simulink model "Heli2DoF"  (R2024b)
settings: Solver=VariableStepAuto  StartTime=0.0  StopTime=30  RelTol=1e-3
values from neighbouring files (symbols this model uses):
  A = [0 0 1 0; 0 0 0 1; pp_ss.A(2,1) 0 pp_ss.A(2,2) 0; 0 0 0 yy_ss.A(2,2)]    [HeliControl.m]    (also in heli.mat = [0 0 -1.26336469915 0 0 0 0 0 1 0 -0.543659539999 0 ... (16 )
  B = [pp_ss.B(1,1) 0; yp_ss.B(1,1) 0; pp_ss.B(2,1) 0; 0 yy_ss.B(2,1)]    [HeliControl.m]    (also in heli.mat = [0.0358066695789  0; 0.0354869266893  0; 0.022302435285  0; )
  C = [1 0 0 0; 0 1 0 0]    [HeliControl.m]    (also in heli.mat = [1  0  0  0; 0  1  0  0])
  K = Ks(:,1:4)    [HeliControl.m]    (also in heli.mat = [45.6610986225  20.6092759277  20.0236061253  7.57450439059;)
  K_q = Kq(:,1:4)    [HeliControl.m]    (also in heli.mat = [20.1841001288  13.9498910139  11.326144531  5.03030863759; )
  Ki = -Ks(:,5:6)    [HeliControl.m]    (also in heli.mat = [18.7111763277  13.9796595605; 21.5110334967  -19.8867838349)
  Ki_q = -Kq(:,5:6)    [HeliControl.m]    (also in heli.mat = [19.1284159126  11.5803153962; 23.1606307923  -38.2568318252)
settings Model: Creator=nagel  LastModifiedBy=nagel

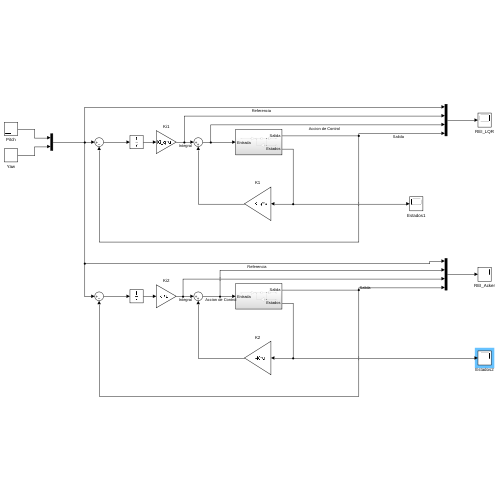
[thumbnail: Simulink's stored preview of the top-level diagram]
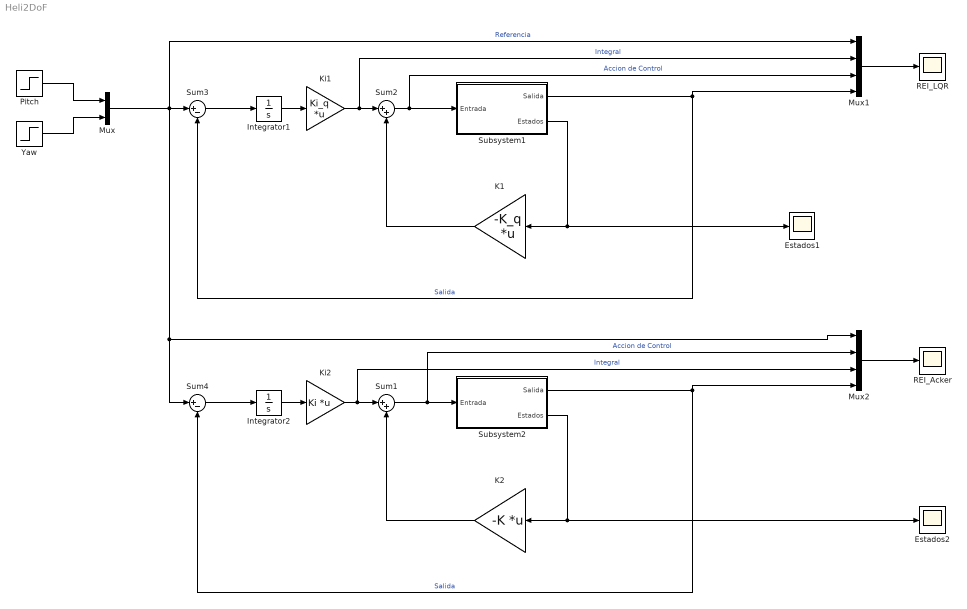
== system Heli2DoF ==
  Estados1 : Scope
  Estados2 : Scope
  Integrator1 : Integrator
  Integrator2 : Integrator
  K1 : Gain  Gain=-K_q  Multiplication=Matrix(K*u)
  K2 : Gain  Gain=-K  Multiplication=Matrix(K*u)
  Ki1 : Gain  Gain=Ki_q  Multiplication=Matrix(K*u)
  Ki2 : Gain  Gain=Ki  Multiplication=Matrix(K*u)
  Mux : Mux  Inputs=2
  Mux1 : Mux
  Mux2 : Mux
  Pitch : Step  Time=0  After=0.583  SampleTime=0
  REI_Acker : Scope
  REI_LQR : Scope
  Subsystem1 : Subsystem
  Subsystem2 : Subsystem
  Sum1 : Sum  Inputs=|++
  Sum2 : Sum  Inputs=|++
  Sum3 : Sum  Inputs=|+-
  Sum4 : Sum  Inputs=|+-
  Yaw : Step  Time=0  After=0  SampleTime=0
  wires:
  Sum3/1 -> Integrator1/1
  Integrator1/1 -> Ki1/1
  Subsystem1/2(Estados) -> Estados1/1, K1/1
  K1/1 -> Sum2/2
  Ki1/1 -> Mux1/2, Sum2/1  "Integral"
  Subsystem1/1(Salida) -> Sum3/2, Mux1/4  "Salida"
  Mux1/1 -> REI_LQR/1
  Sum2/1 -> Subsystem1/1(Entrada), Mux1/3  "Accion de Control"
  Yaw/1 -> Mux/2
  Pitch/1 -> Mux/1
  Ki2/1 -> Mux2/3, Sum1/1  "Integral"
  Mux/1 -> Sum4/1, Mux2/1, Mux1/1, Sum3/1  "Referencia"
  Subsystem2/2(Estados) -> Estados2/1, K2/1
  Sum1/1 -> Mux2/2, Subsystem2/1(Entrada)  "Accion de Control"
  K2/1 -> Sum1/2
  Subsystem2/1(Salida) -> Mux2/4, Sum4/2  "Salida"
  Integrator2/1 -> Ki2/1
  Sum4/1 -> Integrator2/1
  Mux2/1 -> REI_Acker/1

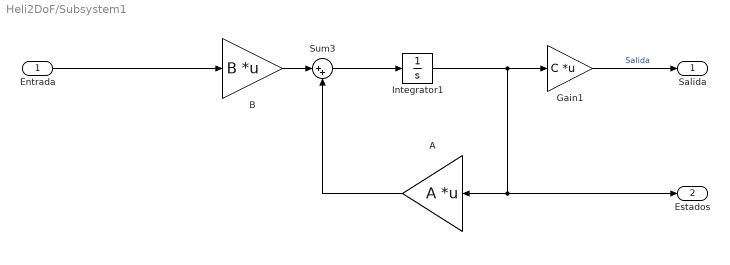
== system Heli2DoF/Subsystem1 ==
  Entrada : Inport
  A : Gain  Gain=A  Multiplication=Matrix(K*u)
  B : Gain  Gain=B  Multiplication=Matrix(K*u)
  Gain1 : Gain  Gain=C  Multiplication=Matrix(K*u)
  Integrator1 : Integrator
  Sum3 : Sum  Inputs=|++
  Salida : Outport
  Estados : Outport  Port=2
  wires:
  Sum3/1 -> Integrator1/1
  B/1 -> Sum3/1
  A/1 -> Sum3/2
  Gain1/1 -> Salida/1  "Salida"
  Integrator1/1 -> A/1, Estados/1, Gain1/1
  Entrada/1 -> B/1

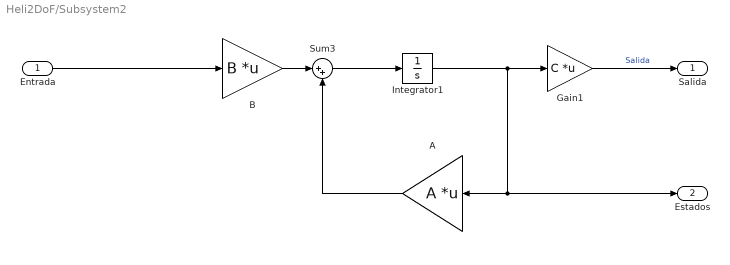
== system Heli2DoF/Subsystem2 ==
  Entrada : Inport
  A : Gain  Gain=A  Multiplication=Matrix(K*u)
  B : Gain  Gain=B  Multiplication=Matrix(K*u)
  Gain1 : Gain  Gain=C  Multiplication=Matrix(K*u)
  Integrator1 : Integrator
  Sum3 : Sum  Inputs=|++
  Salida : Outport
  Estados : Outport  Port=2
  wires:
  Sum3/1 -> Integrator1/1
  B/1 -> Sum3/1
  A/1 -> Sum3/2
  Gain1/1 -> Salida/1  "Salida"
  Integrator1/1 -> A/1, Estados/1, Gain1/1
  Entrada/1 -> B/1
